simulink model "Drone_Flight_Model_StandAlone_KF_Steady"  (R2016b)
settings: Solver=FixedStepDiscrete  StartTime=0.0  StopTime=20  FixedStep=1/400  RelTol=1e-3  EnableMultiTasking=on
model workspace: external: MAT-File C:\Users\Patrick\Documents\TU\Integration project\AR_Drone_Models\Flight_Models\PD\parameters.mat (data not in the file)
undefined symbols (not defined in the file): accelerometerXyzGains, accelerometerXyzOffsets, Ak, Bk, botCamData, Ck, D_height, D_pitch, D_roll, D_yaw, DiscIntNeverNeededParam, Dk, Drone_StateModeType, dronePowerScaling, g, gyroXyzOffsets, I_height, M, magnetoXyzOffsets, Mass, P_height, P_pitch, P_roll, P_yaw, propDistance, yawTorqueC
libraries: simulink x17, dspstat3 x3, AR_Drone_Sensors x3, AR_Drone_Actuators x3, dspnetwork x2, visionanalysis x2, vrlib x2, AR_Drone_Video x1, AR_Drone_Positioning x1
(part 2 of 2)

== system Drone_Flight_Model_StandAlone_KF_Steady/Sensors, Calibration, Raw state computation/IMU Data Acquisition, Validation, Calibration and Initialization/Sensor Initialization ==
  Measurement_Calculation_Bus : Inport
  Drone_StateModeType : Inport  Port=2
  Bus Creator : BusCreator  Inputs=4
  Bus Selector : BusSelector  OutputSignals=UltraSound_Calculation,AccelNorm_Calculation,Gyro_Calculation,Magnetometer_Calculation
  Gyro Offset Initialization : Subsystem
  Signal Specification : SignalSpecification  SampleTime=1/400
  Initalized Measurement_Calculation_Bus : Outport
  wires:
  Bus Selector/2 -> Bus Creator/2  "<AccelNorm_Calculation>"
  Bus Selector/1 -> Bus Creator/1  "<UltraSound_Calculation>"
  Bus Selector/4 -> Bus Creator/4  "<Magnetometer_Calculation>"
  Measurement_Calculation_Bus/1 -> Bus Selector/1
  Bus Selector/3 -> Gyro Offset Initialization/1(Gyro_Calculation)  "<Gyro_Calculation>"
  Drone_StateModeType/1 -> Gyro Offset Initialization/2(Drone_StateModeType)
  Gyro Offset Initialization/1(Initalized Gyro) -> Bus Creator/3
  Signal Specification/1 -> Initalized Measurement_Calculation_Bus/1
  Bus Creator/1 -> Signal Specification/1

== system Drone_Flight_Model_StandAlone_KF_Steady/Take-Off, Landing, Safety, Motor drivers/AR Drone Motors/MotorMixing ==
  altitude_command : Inport
  roll_command : Inport  Port=2
  pitch_command : Inport  Port=3
  yaw_command : Inport  Port=4
  Constant : Constant  Value=100
  Motor input allocation Result is pure forces : Gain  Gain=[1 1/propDistance 1/propDistance -yawTorqueC; 1 -1/propDistance 1/propDistance yawTorqueC; 1 -1/propDistance -1/propDistance -yawTorqueC; 1 1/propDistance -1/propDistance yawTorqueC]  Multiplication=Matrix(K*u)  ParamDataTypeStr=int16
  Mux1 : Mux
  Newton To PWM : MATLAB Function  TreatAsAtomicUnit=on  mask{dronePowerScaling=dronePowerScaling}
      mask prompts: dronePowerScaling "Drone Power Factor"
  Saturation Dynamic : simulink/Discontinuities/Saturation Dynamic  SCDEnableBlockLinearizationSpecification=on  OutMin=[]  OutMax=[]  OutDataTypeStr=Inherit: Same as second input  OutDataType=fixdt(1, 16)  OutScaling=2^-10  DoSatur=off
  throttleMinimum : Constant  Value=0
  MotorCommands : Outport
  wires:
  pitch_command/1 -> Mux1/3
  roll_command/1 -> Mux1/2
  altitude_command/1 -> Mux1/1
  throttleMinimum/1 -> Saturation Dynamic/3
  Constant/1 -> Saturation Dynamic/1
  Saturation Dynamic/1 -> MotorCommands/1  "rightCommand"
  yaw_command/1 -> Mux1/4
  Newton To PWM/1(PWM) -> Saturation Dynamic/2
  Motor input allocation Result is pure forces/1 -> Newton To PWM/1(thrustIn)
  Mux1/1 -> Motor input allocation Result is pure forces/1

== system Drone_Flight_Model_StandAlone_KF_Steady/Take-Off, Landing, Safety, Motor drivers/Landing//TakeOff Sequence Controller/Landing//TakeOff Altitude Control ==
  Drone StateModeType : Inport
  Attitude Hover Control : Inport  Port=2
  Initialize computation Controller : Subsystem
  Landing Controller : Subsystem
  TakeOff Controller : Subsystem
  Attitude Control : Outport
  wires:
  TakeOff Controller/1(Attitude TakeOff Control) -> Initialize computation Controller/1(Attitude Control)
  Attitude Hover Control/1 -> Landing Controller/1(Hover Control)
  Landing Controller/1(Attitude Landing Control) -> TakeOff Controller/1(Attitude Control)
  Drone StateModeType/1 -> Landing Controller/2(Drone StateModeType), TakeOff Controller/2(Drone StateModeType), Initialize computation Controller/2(Drone StateModeType)
  Initialize computation Controller/1(Initialization Control) -> Attitude Control/1

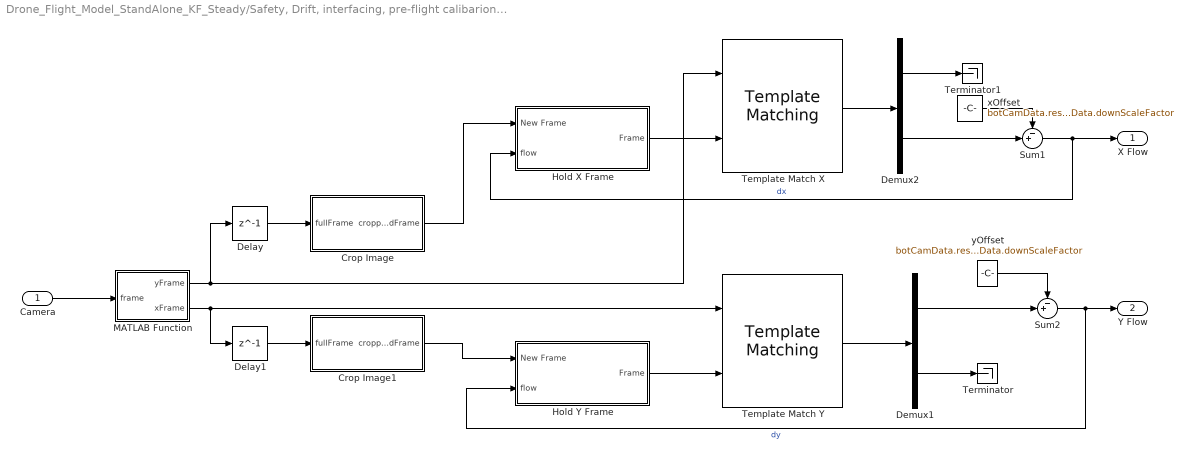
== system Drone_Flight_Model_StandAlone_KF_Steady/Safety, Drift, interfacing, pre-flight calibarion/Optical Flow/Optical Flow/Template Matching ==
  Camera : Inport
  Crop Image : MATLAB Function  TreatAsAtomicUnit=on
  Crop Image1 : MATLAB Function  TreatAsAtomicUnit=on
  Delay : Delay  DelayLength=1
  Delay1 : Delay  DelayLength=1
  Demux1 : Demux  Outputs=2
  Demux2 : Demux  Outputs=2
  Hold X Frame : Subsystem
  Hold Y Frame : Subsystem
  MATLAB Function : MATLAB Function  TreatAsAtomicUnit=on
  Sum1 : Sum  Inputs=-+|  AccumDataTypeStr=double  OutDataTypeStr=double
  Sum2 : Sum  Inputs=-+|  AccumDataTypeStr=double  OutDataTypeStr=double
  Template Match X : visionanalysis/Template Matching  metric=Sum of absolute differences  output=Best match location  method=Three-step  nMetric=off  nSize=3  roi=off  roiValid=off  accumMode=Binary point scaling  accumWordLength=32  accumFracLength=0  prodOutputMode=Binary point scaling  prodOutputWordLength=32  prodOutputFracLength=0  roundingMode=Floor  overflowMode=off
  Template Match Y : visionanalysis/Template Matching  metric=Sum of absolute differences  output=Best match location  method=Three-step  nMetric=off  nSize=3  roi=off  roiValid=off  accumMode=Binary point scaling  accumWordLength=32  accumFracLength=0  prodOutputMode=Binary point scaling  prodOutputWordLength=32  prodOutputFracLength=0  roundingMode=Floor  overflowMode=off
  Terminator : Terminator
  Terminator1 : Terminator
  xOffset : Constant  Value=botCamData.resolution(2)/2/botCamData.downScaleFactor
  yOffset : Constant  Value=botCamData.resolution(1)/2/botCamData.downScaleFactor
  X Flow : Outport
  Y Flow : Outport  Port=2
  wires:
  Demux1/2 -> Terminator/1
  Demux2/1 -> Terminator1/1
  Sum2/1 -> Y Flow/1, Hold Y Frame/2(flow)  "dy"
  Hold Y Frame/1(Frame) -> Template Match Y/2
  Demux1/1 -> Sum2/2
  Template Match Y/1 -> Demux1/1
  MATLAB Function/1(yFrame) -> Template Match X/1, Delay/1
  Delay/1 -> Crop Image/1(fullFrame)
  yOffset/1 -> Sum2/1
  Crop Image/1(croppedFrame) -> Hold X Frame/1(New Frame)
  xOffset/1 -> Sum1/1
  Demux2/2 -> Sum1/2
  Template Match X/1 -> Demux2/1
  Hold X Frame/1(Frame) -> Template Match X/2
  Sum1/1 -> X Flow/1, Hold X Frame/2(flow)  "dx"
  Camera/1 -> MATLAB Function/1(frame)
  Delay1/1 -> Crop Image1/1(fullFrame)
  MATLAB Function/2(xFrame) -> Delay1/1, Template Match Y/1
  Crop Image1/1(croppedFrame) -> Hold Y Frame/1(New Frame)

== system Drone_Flight_Model_StandAlone_KF_Steady/Safety, Drift, interfacing, pre-flight calibarion/Optical Flow/Optical Flow Reset/Drone_StateMode Reset Condition ==
  Drone_StateMode : Inport
  Enumerated Constant2 : simulink/Sources/Enumerated Constant  OutDataTypeStr=Enum: Drone_StateModeType  Value=Drone_StateModeType.Drift_Compensated_Flight  SampleTime=inf
      settings: AttributesFormatString=%<Value>
  Offset Calc Reset Boolean : RelationalOperator  Operator=~=  OutDataTypeStr=boolean  RndMeth=Nearest
  Drone_StateMode Reset : Outport
  wires:
  Drone_StateMode/1 -> Offset Calc Reset Boolean/1
  Enumerated Constant2/1 -> Offset Calc Reset Boolean/2
  Offset Calc Reset Boolean/1 -> Drone_StateMode Reset/1

== system Drone_Flight_Model_StandAlone_KF_Steady/Safety, Drift, interfacing, pre-flight calibarion/Optical Flow/Optical Flow Reset/PQR Reset Condition ==
  PQR : Inport
  Abs : Abs
  Demux : Demux  Outputs=3
  Logical Operator : Logic  Operator=OR  Inputs=3  AllPortsSameDT=off  OutDataTypeStr=boolean
  Max P : simulink/Logic and Bit Operations/Compare To Constant  relop=>  const=30  OutDataTypeStr=uint8
  Max Q : simulink/Logic and Bit Operations/Compare To Constant  relop=>  const=30  OutDataTypeStr=uint8
  Max R : simulink/Logic and Bit Operations/Compare To Constant  relop=>  const=30  OutDataTypeStr=uint8
  PQR Reset : Outport
  wires:
  Demux/1 -> Max P/1
  Demux/2 -> Max Q/1
  Max P/1 -> Logical Operator/1
  Max Q/1 -> Logical Operator/2
  Logical Operator/1 -> PQR Reset/1
  Demux/3 -> Max R/1
  Max R/1 -> Logical Operator/3
  Abs/1 -> Demux/1
  PQR/1 -> Abs/1

== system Drone_Flight_Model_StandAlone_KF_Steady/Safety, Drift, interfacing, pre-flight calibarion/Optical Flow/Optical Flow Reset/Zdot Reset condition ==
  Z Zdot : Inport
  Abs : Abs
  Demux : Demux  Outputs=2
  Max Zdot : simulink/Logic and Bit Operations/Compare To Constant  relop=>  const=20  OutDataTypeStr=uint8
  Smooth Height : DiscreteTransferFcn  Numerator=[0.05]  Denominator=[1 -0.95]
  Terminator : Terminator
  Zdot Reset : Outport
  wires:
  Max Zdot/1 -> Zdot Reset/1
  Z Zdot/1 -> Demux/1
  Abs/1 -> Smooth Height/1
  Demux/1 -> Terminator/1
  Demux/2 -> Abs/1
  Smooth Height/1 -> Max Zdot/1

== system Drone_Flight_Model_StandAlone_KF_Steady/Sensors, Calibration, Raw state computation/IMU Data Acquisition, Validation, Calibration and Initialization/Measurement Verification and Calibration/Measurement calibration correction ==
  note: Cannot measure below ~15cm so it is set as minimum
  MeasurementDataBus : Inport
  Accelerometer calibration : Subsystem
  Bus Creator1 : BusCreator  Inputs=4
  Bus Selector : BusSelector  OutputSignals=Ultrasound_Measure,Accelerometer_Measure,BodyRates_Measure,Magnetometer_Measure
  Calibration_Scale_and_Offset1 : Subsystem
  Gyro offset : Subsystem
  Height Lookup Table : Lookup_n-D  NumberOfTableDimensions=1  BreakpointsForDimension1="[880\t896.633239612621\t926.474851608872\t963.444876423216\t1026.24093976506\t1108.89023120183\t1201.82715535194\t1299.73045340950\t1400.50546704155\t1505.69346105789\t1616.54602249063\t1723.41949303820\t1829.85256143274\t1941.57919400187\t2209.22354901416\t2928.85067166510\t3648.07466416745\t4365.64658835291\t5080.81671757845\t5793.22994251437\t6544.72960690752\t7259.40674789128\t8002\t8664.09897525619\t9309.60334916271\t9993]"  Table="[15\t20\t23\t26\t29\t32\t35\t38\t41\t44\t47\t50\t53\t56\t63\t83\t103\t123\t143\t163\t183\t203\t223\t243\t263\t283]"  InternalRulePriority=Speed  RndMeth=Simplest  InputSameDT=on
  MATLAB Function : MATLAB Function  TreatAsAtomicUnit=on
  Measurement_Calculation_Bus : Outport
  wires:
  Bus Selector/1 -> MATLAB Function/1(Ultrasound_Measure)  "<Ultrasound_Measure>"
  Gyro offset/1(Gyro Offset Remove) -> Bus Creator1/3  "Gyro_Calculation"
  Bus Selector/2 -> Accelerometer calibration/1(Accel)  "<Accelerometer_Measure>"
  Accelerometer calibration/1(Accel_Norm) -> Bus Creator1/2  "AccelNorm_Calculation"
  Height Lookup Table/1 -> Bus Creator1/1  "UltraSound_Calculation"
  Calibration_Scale_and_Offset1/1(Normalized  Magnetometer) -> Bus Creator1/4  "Magnetometer_Calculation"
  MeasurementDataBus/1 -> Bus Selector/1
  Bus Selector/3 -> Gyro offset/1(Raw Gyro Values)  "<BodyRates_Measure>"
  Bus Creator1/1 -> Measurement_Calculation_Bus/1
  Bus Selector/4 -> Calibration_Scale_and_Offset1/1(RawMag)  "<Magnetometer_Measure>"
  MATLAB Function/1(processed_Ultrasound) -> Height Lookup Table/1  "UltraSound_Calculation"

== system Drone_Flight_Model_StandAlone_KF_Steady/Sensors, Calibration, Raw state computation/IMU Data Acquisition, Validation, Calibration and Initialization/Sensor Initialization/Gyro Offset Initialization ==
  note: Gyro Offset Initialization
      | The gyro is calibrated each time before flight takes place during the
      | Drone_StateModeType.Initialize state. The gyro is the only sensor that
      | can be re calibrated from the static take off position.
  Gyro_Calculation : Inport
  Drone_StateModeType : Inport  Port=2
  Add : Sum  Inputs=+-
  Compute Gyro Offset : dspstat3/Mean  run=on  reset_popup=Rising edge  directionMode=Each column  dimension=1  roiEnable=off  roiType=Rectangles  roiPortion=Entire ROI  roiOutput=Individual statistics for each ROI  roiFlag=off  outputDataTypeStr=Inherit: Same as accumulator  outputLastDataTypeStr=Inherit: Same as accumulator  outputMin=[]  outputMax=[]  roundingMode=Floor  overflowMode=off
  Enumerated Constant2 : simulink/Sources/Enumerated Constant  OutDataTypeStr=Enum: Drone_StateModeType  Value=Drone_StateModeType.Initialize_Sensors  SampleTime=inf
      settings: AttributesFormatString=%<Value>
  Offset Calc Reset Boolean : RelationalOperator  Operator===  OutDataTypeStr=boolean  RndMeth=Nearest
  Offset Memory : Memory  InheritSampleTime=on
  Output Selector : Switch  Criteria=u2 > Threshold
  Output Selector Reset Boolean : RelationalOperator  Operator=~=  OutDataTypeStr=boolean  RndMeth=Nearest
  Initalized Gyro : Outport
  wires:
  Offset Calc Reset Boolean/1 -> Compute Gyro Offset/2
  Gyro_Calculation/1 -> Add/1, Compute Gyro Offset/1
  Output Selector Reset Boolean/1 -> Output Selector/2
  Compute Gyro Offset/1 -> Output Selector/3
  Output Selector/1 -> Offset Memory/1, Add/2
  Add/1 -> Initalized Gyro/1  "Gyro_Calculation"
  Drone_StateModeType/1 -> Output Selector Reset Boolean/2, Offset Calc Reset Boolean/2
  Offset Memory/1 -> Output Selector/1
  Enumerated Constant2/1 -> Output Selector Reset Boolean/1, Offset Calc Reset Boolean/1

== system Drone_Flight_Model_StandAlone_KF_Steady/Take-Off, Landing, Safety, Motor drivers/Landing//TakeOff Sequence Controller/Landing//TakeOff Altitude Control/Initialize computation Controller ==
  note: Magnetometer initialization controls
      | The motors influence the magnetometer measurement.
      | The motors are set to turn at low RPM while computing the yaw offset.
  Attitude Control : Inport
  Drone StateModeType : Inport  Port=2
  Enumerated Constant2 : simulink/Sources/Enumerated Constant  OutDataTypeStr=Enum: Drone_StateModeType  Value=Drone_StateModeType.Initialize_Computation  SampleTime=inf
      settings: AttributesFormatString=%<Value>
  Initialize Boolean : RelationalOperator  Operator=~=  OutDataTypeStr=boolean  RndMeth=Nearest
  Magneto initialization thrust : Constant  Value="Mass * 9.81 * 0.15  / 4"
  Switch2 : Switch  Criteria=u2 > Threshold
  Initialization Control : Outport
  wires:
  Enumerated Constant2/1 -> Initialize Boolean/1
  Drone StateModeType/1 -> Initialize Boolean/2
  Attitude Control/1 -> Switch2/1
  Initialize Boolean/1 -> Switch2/2
  Switch2/1 -> Initialization Control/1
  Magneto initialization thrust/1 -> Switch2/3

== system Drone_Flight_Model_StandAlone_KF_Steady/Take-Off, Landing, Safety, Motor drivers/Landing//TakeOff Sequence Controller/Landing//TakeOff Altitude Control/Landing Controller ==
  note: Landing Sequence control
      | The last known altitude PWM signal is decayed such that the drone loses altitude controlled.
  Hover Control : Inport
  Drone StateModeType : Inport  Port=2
  Decay Gain : Gain  Gain=0.9992
  Enumerated Constant1 : simulink/Sources/Enumerated Constant  OutDataTypeStr=Enum: Drone_StateModeType  Value=Drone_StateModeType.Landing_RampDown  SampleTime=inf
      settings: AttributesFormatString=%<Value>
  Landing Boolean : RelationalOperator  Operator=~=  OutDataTypeStr=boolean  RndMeth=Nearest
  Memory : Memory
  Switch1 : Switch  Criteria=u2 > Threshold
  Attitude Landing Control : Outport
  wires:
  Memory/1 -> Decay Gain/1
  Landing Boolean/1 -> Switch1/2
  Decay Gain/1 -> Switch1/3
  Enumerated Constant1/1 -> Landing Boolean/1
  Hover Control/1 -> Switch1/1
  Switch1/1 -> Memory/1, Attitude Landing Control/1
  Drone StateModeType/1 -> Landing Boolean/2

== system Drone_Flight_Model_StandAlone_KF_Steady/Take-Off, Landing, Safety, Motor drivers/Landing//TakeOff Sequence Controller/Landing//TakeOff Altitude Control/TakeOff Controller ==
  note: Take Off control
      | The altitude PWM signal is ramped up from a bottom value to a maximum of 45% of hover thrust before
      | height control is enabled.
  Attitude Control : Inport
  Drone StateModeType : Inport  Port=2
  Base Required Thrust Per Motor [N] : Constant  Value=Mass * 9.81 * 0.45 / 4
  Discrete-Time Integrator : DiscreteIntegrator  gainval=1  ExternalReset=level  InitialConditionSource=external  InitialConditionSetting=State (most efficient)  SampleTime=-1  ICPrevOutput=DiscIntNeverNeededParam  ICPrevScaledInput=DiscIntNeverNeededParam
  Enumerated Constant2 : simulink/Sources/Enumerated Constant  OutDataTypeStr=Enum: Drone_StateModeType  Value=Drone_StateModeType.Take_Off  SampleTime=inf
      settings: AttributesFormatString=%<Value>
  Initial Thrust value : Constant  Value="Mass * 9.81 * 0.2  / 4"
  Saturation : Saturate  UpperLimit=0.5*Mass * 9.81 / 4  LowerLimit=0
  Switch2 : Switch  Criteria=u2 > Threshold
  TakeOff Boolean : RelationalOperator  Operator=~=  OutDataTypeStr=boolean  RndMeth=Nearest
  Attitude TakeOff Control : Outport
  wires:
  Enumerated Constant2/1 -> TakeOff Boolean/1
  Saturation/1 -> Switch2/3
  Drone StateModeType/1 -> TakeOff Boolean/2
  Attitude Control/1 -> Switch2/1
  TakeOff Boolean/1 -> Switch2/2, Discrete-Time Integrator/2
  Switch2/1 -> Attitude TakeOff Control/1
  Discrete-Time Integrator/1 -> Saturation/1
  Base Required Thrust Per Motor [N]/1 -> Discrete-Time Integrator/1
  Initial Thrust value/1 -> Discrete-Time Integrator/3

== system Drone_Flight_Model_StandAlone_KF_Steady/Safety, Drift, interfacing, pre-flight calibarion/Optical Flow/Optical Flow/Template Matching/Hold X Frame ==
  New Frame : Inport
  flow : Inport  Port=2
  Delay2 : Delay  DelayLength=1  InitialConditionSource=Input port
      settings: InputPortMap=u0,p4
  Delay3 : Delay  DelayLength=1
  MATLAB Function : MATLAB Function  TreatAsAtomicUnit=on
  Frame : Outport
  wires:
  Delay2/1 -> MATLAB Function/2(heldFrame)
  MATLAB Function/1(referenceFrame) -> Delay2/1, Frame/1
  New Frame/1 -> MATLAB Function/1(currentFrame), Delay2/2
  flow/1 -> Delay3/1
  Delay3/1 -> MATLAB Function/3(flow)

== system Drone_Flight_Model_StandAlone_KF_Steady/Safety, Drift, interfacing, pre-flight calibarion/Optical Flow/Optical Flow/Template Matching/Hold Y Frame ==
  New Frame : Inport
  flow : Inport  Port=2
  Delay2 : Delay  DelayLength=1  InitialConditionSource=Input port
      settings: InputPortMap=u0,p4
  Delay3 : Delay  DelayLength=1
  MATLAB Function : MATLAB Function  TreatAsAtomicUnit=on
  Frame : Outport
  wires:
  Delay2/1 -> MATLAB Function/2(heldFrame)
  MATLAB Function/1(referenceFrame) -> Delay2/1, Frame/1
  New Frame/1 -> MATLAB Function/1(currentFrame), Delay2/2
  flow/1 -> Delay3/1
  Delay3/1 -> MATLAB Function/3(flow)

== system Drone_Flight_Model_StandAlone_KF_Steady/Sensors, Calibration, Raw state computation/IMU Data Acquisition, Validation, Calibration and Initialization/Measurement Verification and Calibration/Measurement calibration correction/Accelerometer calibration ==
  Accel : Inport
  Apply calibration parameters : Subsystem
  Data Type Conversion : DataTypeConversion  OutDataTypeStr=double
  Normalize Vector : vrlib/Utilities/Normalize Vector  Commented=through  maxzero=0
  Accel_Norm : Outport
  wires:
  Accel/1 -> Data Type Conversion/1
  Data Type Conversion/1 -> Apply calibration parameters/1(Raw Accelerometer Data)
  Normalize Vector/1 -> Accel_Norm/1
  Apply calibration parameters/1(Calibrated Accelerometer Data) -> Normalize Vector/1

== system Drone_Flight_Model_StandAlone_KF_Steady/Sensors, Calibration, Raw state computation/IMU Data Acquisition, Validation, Calibration and Initialization/Measurement Verification and Calibration/Measurement calibration correction/Calibration_Scale_and_Offset1 ==
  RawMag : Inport
  Add : Sum  Inputs=-+
  Constant : Constant  Value=magnetoXyzOffsets
  Normalize Vector : vrlib/Utilities/Normalize Vector  maxzero=0
  Normalized  Magnetometer : Outport
  wires:
  Add/1 -> Normalize Vector/1
  Constant/1 -> Add/1
  Normalize Vector/1 -> Normalized  Magnetometer/1
  RawMag/1 -> Add/2

== system Drone_Flight_Model_StandAlone_KF_Steady/Sensors, Calibration, Raw state computation/IMU Data Acquisition, Validation, Calibration and Initialization/Measurement Verification and Calibration/Measurement calibration correction/Gyro offset ==
  Raw Gyro Values : Inport
  Constant : Constant  Value=gyroXyzOffsets  VectorParams1D=off
  Demux : Demux  Outputs=3
  Demux1 : Demux  Outputs=3
  Mux1 : Mux  Inputs=3
  Process Raw Rate Gyro Data : Subsystem
  Sum : Sum  Inputs=|+-
  Sum1 : Sum  Inputs=|+-
  Sum2 : Sum  Inputs=|+-
  Gyro Offset Remove : Outport
  wires:
  Demux/3 -> Sum2/1
  Sum1/1 -> Mux1/2
  Demux1/1 -> Sum/2
  Sum2/1 -> Mux1/3
  Demux/2 -> Sum1/1
  Demux/1 -> Sum/1
  Sum/1 -> Mux1/1
  Mux1/1 -> Process Raw Rate Gyro Data/1(Raw Rate Gyro Data)
  Demux1/2 -> Sum1/2
  Demux1/3 -> Sum2/2
  Process Raw Rate Gyro Data/1(Processed Data) -> Gyro Offset Remove/1
  Constant/1 -> Demux1/1
  Raw Gyro Values/1 -> Demux/1

== system Drone_Flight_Model_StandAlone_KF_Steady/Sensors, Calibration, Raw state computation/IMU Data Acquisition, Validation, Calibration and Initialization/Measurement Verification and Calibration/Measurement calibration correction/Accelerometer calibration/Apply calibration parameters ==
  Raw Accelerometer Data : Inport
  Acclerometer Calibration Gains : Constant  Value=accelerometerXyzGains
  Acclerometer Calibration Offsets : Constant  Value=accelerometerXyzOffsets
  Add : Sum  Inputs=+-
  Divide : Product  Inputs=*/
  Calibrated Accelerometer Data : Outport
  wires:
  Divide/1 -> Calibrated Accelerometer Data/1
  Raw Accelerometer Data/1 -> Add/1
  Acclerometer Calibration Gains/1 -> Divide/2
  Acclerometer Calibration Offsets/1 -> Add/2
  Add/1 -> Divide/1

== system Drone_Flight_Model_StandAlone_KF_Steady/Sensors, Calibration, Raw state computation/IMU Data Acquisition, Validation, Calibration and Initialization/Measurement Verification and Calibration/Measurement calibration correction/Gyro offset/Process Raw Rate Gyro Data ==
  note: const float Sensitivity[ 3 ] = { 0.0609 , 0.0609 , 0.0609 } ;
  Raw Rate Gyro Data : Inport
  Flip Pitch Yaw Direction For Calculation #235 : Gain  Gain=[1 -1 -1]
  Gain : Gain  Gain=[0.0609, 0.0609, 0.0609]  ParamDataTypeStr=double
  Processed Data : Outport
  wires:
  Raw Rate Gyro Data/1 -> Gain/1
  Flip Pitch Yaw Direction For Calculation #235/1 -> Processed Data/1
  Gain/1 -> Flip Pitch Yaw Direction For Calculation #235/1

== matlab function Drone_Flight_Model_StandAlone_KF_Steady/Safety, Drift, interfacing, pre-flight calibarion/Downscaled Bottom Camera/Downscale Chroma Image ==
  data: YCbCr422In input; cameraChroma output; width parameter; height parameter; downScaleFactor parameter
function cameraChroma    = downscaleY(YCbCr422In,width, height, downScaleFactor)
 
cameraChroma = uint8(zeros(height/downScaleFactor,width/downScaleFactor));
if ~isempty(YCbCr422In)

    %% Downsample and keep only the chromatic value

    for verticalIndex = 1 : 1 : height/downScaleFactor;             % indexing for downsampled vertical direction
        for horizontalIndex = 1 : 1 : (width / 2)/downScaleFactor;  % indexing for downsampled horizontal direction
            index = 4 * (downScaleFactor * (verticalIndex - 1) * (width / 2) + downScaleFactor * horizontalIndex) - 3;  % translate the horizontal and vertical indexes into the index into the video input
            cameraChroma(verticalIndex, 2 * horizontalIndex - [1 0]) = [YCbCr422In(index+1) YCbCr422In(index+3)];
        end
    end
end
end

== matlab function Drone_Flight_Model_StandAlone_KF_Steady/Safety, Drift, interfacing, pre-flight calibarion/Optical Flow/Optical Flow/Template Matching/Crop Image ==
  data: fullFrame input; croppedFrame output
function croppedFrame = CropImage(fullFrame)

%% Template matching works by pixel shifting a smaller image within the full image
% Exhaustive template matching will compute all possible pixel shifts.
% Because of this the cropAmount influences the computation time
% quadratically. A small crop amount increases the computation speed but
% also limits the maximum detectable pixel shift between frames. 
% Three step template matching also has increasing computational time with
% increasing cropAmount, but much less so than the exhaustive method.
cropAmount = 7;
%% Maximizing camera FPS
% Doubling the camera FPS doubles the computation time but also means you 
% can halve the cropAmount and still detect the same velocity range, which 
% reduces the computational time up to a factor 4.
%% FPS limitations
% Using a very high fps means that slow drone movements will not lead to
% significant enough displacement between images. This means that slow
% drift is not detected. Holding the reference frame untill movement is
% deteced is a way around this.


[row, col] = size(fullFrame);
croppedFrame = fullFrame(1 + cropAmount : row - cropAmount, 1 + cropAmount : col - cropAmount);
% croppedFrame = fullFrame(1 + cropAmount : row - cropAmount, 1 : col);

== stateflow chart Drone_Flight_Model_StandAlone_KF_Steady/Safety, Drift, interfacing, pre-flight calibarion/Supervisory Flight Controller ==
  state stateChecks [parallel]
    settings: executionOrder=1
    note: Description:
        | This state containts the sub states used to detect specific operating conditions
    state batteryFaultCheck [parallel]
      settings: executionOrder=1
      note: Description:
          | This state will indicate whether the battery has enough voltage.
      state batteryNominal
      state batteryLow
      batteryLow -> batteryNominal : [Measured_Battery_Voltage>=10.6]
      batteryNominal -> batteryLow : [Measured_Battery_Voltage<10.6]
      (default) -> batteryLow
    state orientationFaultCheck [parallel]
      settings: executionOrder=2
      note: Description:
          | This state will indicate whether the drone is in a safe orientation
      state nominalOrientation
      state unsafeOrientation
      unsafeOrientation -> nominalOrientation : [all(abs(Euler_Angles(1:2)) < 35)]
      nominalOrientation -> unsafeOrientation : [any(abs(Euler_Angles(1:2)) >= 35)]
      (default) -> unsafeOrientation
    state safeHeightCheck [parallel]
      settings: executionOrder=3
      note: Description:
          | This state will indicate whether the drone is close enough to the groudn for the final landing procedure
      state safeLandingHeight
      state unsafeLandingHeight
      unsafeLandingHeight -> safeLandingHeight : [Altitude < 25]
      safeLandingHeight -> unsafeLandingHeight : [Altitude > 30]
      (default) -> unsafeLandingHeight
  state Drone_State [parallel]
    settings: executionOrder=2
    note: Description:
        | This state contains the logic governing the drone behaviour based on user input and drone state checks
    state WaitForHost
    state Initialize_Sensors
    state Initialize_Computation
    state Take_Off
    state Drift_Compensated_Flight
    state Landing_Terminate
    state Landing_RampDown
    state Landing_Descent
    (default) -> WaitForHost
    Landing_Terminate -> WaitForHost : [ (hostCmd == Drone_StateModeType.WaitForHost)]
    WaitForHost -> Initialize_Sensors : [ (hostCmd == Drone_StateModeType.Drift_Compensated_Flight)...
        | && in(stateChecks.batteryFaultCheck.batteryNominal)...
        | && in (stateChecks.orientationFaultCheck.nominalOrientation)...
        | && after(1.5,sec)]
    Initialize_Sensors -> Initialize_Computation : [after(0.5,sec)]
    Initialize_Computation -> Take_Off : [after(3,sec)]
    Take_Off -> Landing_Terminate [order 2] : [(hostCmd == Drone_StateModeType.Landing_Terminate)]
    Take_Off -> Drift_Compensated_Flight [order 1] : [after(2,sec)]
    Drift_Compensated_Flight -> Landing_Descent [order 1] : [(hostCmd == Drone_StateModeType.Landing_Descent)...
        | ||in(stateChecks.batteryFaultCheck.batteryLow) ]
    Drift_Compensated_Flight -> Landing_Terminate [order 2] : [in(stateChecks.orientationFaultCheck.unsafeOrientation)...
        | ||(hostCmd == Drone_StateModeType.Landing_Terminate)]
    Landing_RampDown -> Landing_Terminate : [after(2.0,sec)...
        | ||(hostCmd == Drone_StateModeType.Landing_Terminate)]
    Landing_Descent -> Landing_RampDown [order 1] : [in(stateChecks.safeHeightCheck.safeLandingHeight)]
    Landing_Descent -> Landing_Terminate [order 2] : [(hostCmd == Drone_StateModeType.Landing_Terminate)]
  data: hostCmd input Enum: Drone_StateModeType; Drone_StateMode output Enum: Drone_StateModeType; Measured_Battery_Voltage input; Euler_Angles input; Altitude input
  data hostCmd settings: description=|
      | The hostCmd can take the values 0,1 and 2.
      | 
      | 0 - default state when the drone is powered up.
      | 1 - Takeoff
      | 2 - Landing

== matlab function Drone_Flight_Model_StandAlone_KF_Steady/Safety, Drift, interfacing, pre-flight calibarion/Drone TO PC UDP IO/Gather Data and transfer rates/MATLAB Function1 ==
  data: dataIn input; combinedData output
function combinedData = combineMultipleSamples(dataIn)

persistent storedData
if isempty(storedData)
    storedData = zeros(66,1);
end
storedData(1:33) = storedData(34:66);
storedData(34:66) = dataIn;
combinedData = storedData;

== matlab function Drone_Flight_Model_StandAlone_KF_Steady/Sensors, Calibration, Raw state computation/Unwrap Yaw Angle/MATLAB Function ==
  data: wrappedYaw input; unwrappedYaw output; previousYaw input
function unwrappedYaw = unwrapYaw(wrappedYaw, previousYaw)
%#codegen

persistent offset
if isempty(offset)
   offset = 0; 
end

threshold = 150;

% check if the yaw switched from ~180 to ~-180
if (previousYaw > threshold && wrappedYaw < -threshold)
    offset = offset + 360;
end

% check if the yaw switched from ~-180 to ~180
if (previousYaw < -threshold && wrappedYaw > threshold)
    offset = offset - 360;
end

unwrappedYaw = wrappedYaw + offset;

== matlab function Drone_Flight_Model_StandAlone_KF_Steady/Controller/Zdot transform/Rotation matrix/Rotm in euler ==
  data: alpha input size=3,1; Rbv output size=3,3
function Rbv = fcn(alpha)
Rbv = [1,0,0;0,cos(alpha(1)),sin(alpha(1));0,-sin(alpha(1)),cos(alpha(1))]*...
      [cos(alpha(2)),0,-sin(alpha(2));0,1,0;sin(alpha(2)),0,cos(alpha(2))]*...
      [cos(alpha(3)),sin(alpha(3)),0;-sin(alpha(3)),cos(alpha(3)),0;0,0,1];

== matlab function Drone_Flight_Model_StandAlone_KF_Steady/Sensors, Calibration, Raw state computation/Calculate Roll Pitch/MATLAB Function ==
  data: Ax_Ay_Az input; Roll output; Pitch output
function [Roll,Pitch] = CalculateAngle(Ax_Ay_Az)

Pitch = atan( Ax_Ay_Az(1) / sqrt( Ax_Ay_Az(2)^2 + Ax_Ay_Az(3)^2));
Roll = atan( Ax_Ay_Az(2) / sqrt( Ax_Ay_Az(1)^2 + Ax_Ay_Az(3)^2));

== matlab function Drone_Flight_Model_StandAlone_KF_Steady/Safety, Drift, interfacing, pre-flight calibarion/Optical Flow/Optical Flow/Template Matching/MATLAB Function ==
  data: yFrame output; frame input; xFrame output
function [yFrame, xFrame] = downSampleFrames(frame)

xFrame = frame(1:4:end,:);
yFrame = frame(:,1:4:end);

== matlab function Drone_Flight_Model_StandAlone_KF_Steady/Safety, Drift, interfacing, pre-flight calibarion/Optical Flow/Optical Flow/Template Matching/Hold Y Frame/MATLAB Function ==
  data: currentFrame input uint8; referenceFrame output; heldFrame input uint8; flow input
function referenceFrame  = holdFrame(currentFrame,heldFrame,flow)

%% This MATLAB function block holds the T frame untill movement is detected
% If the T frame were updated every step, slow movements would not be
% registered. By holding the frame movement can be measured over multiple
% frames.

if (flow ==0)
    referenceFrame = heldFrame;
else
    referenceFrame = currentFrame;
end

== matlab function Drone_Flight_Model_StandAlone_KF_Steady/Safety, Drift, interfacing, pre-flight calibarion/Optical Flow/Optical Flow/Scale Optical Flow Steps ==
  data: xFlow input; xPos output; yFlow input; zPos input; yPos output; downScaleFactor parameter; FOV parameter
function [xPos, yPos] = scaleOpticalFlow(xFlow,yFlow,zPos,downScaleFactor,FOV)
xFOV = FOV * 0.75 / 180 * pi;
yFOV = FOV / 180 * pi;

% prevent division by zero when zPos = 0 -> xMax,xMin,yMax,yMin = 0
if zPos > 0 
    xMin = - tan(xFOV/2) * zPos;
    xMax = tan(xFOV/2) * zPos;
    yMin = - tan(yFOV/2) * zPos;
    yMax = tan(yFOV/2) * zPos;

    xResolution = 240/downScaleFactor;
    yResolution = 320/downScaleFactor;

    %determine how many real world cm one camera pixel is
    xScale = xResolution / (xMax - xMin);
    yScale = yResolution / (yMax - yMin);
    
    %scale the optical flow components
    xPos = xFlow / xScale;
    yPos = - yFlow / yScale; % direction is reversed

else
   xPos = 0;
   yPos = 0;
end

== matlab function Drone_Flight_Model_StandAlone_KF_Steady/Sensors, Calibration, Raw state computation/Compute Yaw ==
  data: Roll input; Pitch input; Magneto input; Yaw output
function Yaw = computeYaw(Roll, Pitch, Magneto)

% convert to rad for calculation
Roll = Roll / 360 * 2 * pi;
Pitch = Pitch / 360 * 2 * pi;

% Applications of Magnetic Sensors for Low Cost Compass Systems, Michael J. Caruso, Honeywell, SSEC.
% Magneto(3) sign is switched as we define the z axis as positive up.

var1 = Magneto(2)*cos(Roll)-Magneto(3)*sin(Roll);
var2 = Magneto(1)*cos(Pitch)+Magneto(2)*sin(Pitch)*sin(Roll)+Magneto(3)*cos(Roll)*sin(Pitch);

% scale to [-180 180] deg
Yaw = - atan2(var1,var2) * 180 / pi;

== matlab function Drone_Flight_Model_StandAlone_KF_Steady/Safety, Drift, interfacing, pre-flight calibarion/Drone TO PC UDP IO/Gather Data and transfer rates/Encode Outgoing Packets ==
  data: droneStateMode input; message output; batteryLevel input; roll input; pitch input; yaw input; altitude input; motorCmd input; flags input
function message = packageEncode(droneStateMode, batteryLevel, roll, pitch, yaw, altitude, motorCmd, flags)

persistent checksum
if isempty(checksum)
    checksum = uint8(0);
end

%% Generate a tick/checksum

if checksum < uint8(255)
    checksum = uint8(checksum + 1);
else
    checksum  = uint8(0);
end

%% The message format is:
% Checksum          uint8[1]
% BatterlyLevel     single[1] cast as uint8[4] 
% DroneStateMode    DroneStateModeType[1] cast as uint8[1]
% Roll              single[1] cast as uint8[4] 
% Pitch             single[1] cast as uint8[4] 
% Yaw               single[1] cast as uint8[4] 
% Altitude          single[1] cast as uint8[4] 
% Motor             single[4] cast as uint8[16]
% chkSum&Reset flag uint8[2]
% Target data       single[15] cast as uint8[60]
% Extra data        single[1] cast as uint8[4] 

%% Cast data to a single before typecasting to uint8
stateModeMessage = uint8(droneStateMode);
batteryMessage = typecast(single(batteryLevel),'uint8');
rollMessage = typecast(single(roll),'uint8');
pitchMessage = typecast(single(pitch),'uint8');
yawMessage = typecast(single(yaw),'uint8');
altitudeMessage = typecast(single(altitude),'uint8');
motorMessage = typecast(single(motorCmd),'uint8');
flagsMessage = uint8(flags);


%% Combine into a message
message = uint8(zeros(1,40));
message(1) = checksum;
message(2:5) = batteryMessage;
message(6) = stateModeMessage;
message(7:10) = rollMessage;
message(11:14) = pitchMessage;
message(15:18) = yawMessage;
message(19:22) = altitudeMessage;
message(23:38) = motorMessage;
message(39:40) = flagsMessage;
% message = [checksum batteryMessage stateModeMessage dataMessage];

== matlab function Drone_Flight_Model_StandAlone_KF_Steady/Safety, Drift, interfacing, pre-flight calibarion/Drone TO PC UDP IO/Decode Incoming Packets ==
  data: message input; length input; userCommand output Enum: Drone_StateModeType; maxUpdateDelay parameter; ledColor output; enableTracking output; remoteControl output; trimCommands output
function [userCommand, ledColor, enableTracking, remoteControl, trimCommands]  = packageDecode(message, length, maxUpdateDelay)

persistent lastReceivedTick updatesSinceLastTick ledCounter lastUserCommand savedTrimCommands savedEnableTracking;
if isempty(lastReceivedTick) || isempty(updatesSinceLastTick) || isempty(ledCounter) ...
       || isempty(lastUserCommand) || isempty(savedTrimCommands)
    lastReceivedTick = 0;
    updatesSinceLastTick = 0;
    ledCounter = 0;
    %% Initial state = WaitForHost
    lastUserCommand = Drone_StateModeType(1);
    savedTrimCommands = int8([0 0]);
    savedEnableTracking = uint8(0);
end;

% default return: use last user command
userCommand = lastUserCommand;
ledColor = 2;
enableTracking = savedEnableTracking;
remoteControl = uint8(0);
trimCommands = savedTrimCommands;

% check if a message is received
if length == 6
   % decode message
   newTick = double(message(1));
   newUserCommand = Drone_StateModeType(message(2));
   enableTracking = message(3);
   remoteControl = message(4);
   trimCommands(1) = typecast(message(5),'int8');
   trimCommands(2) = typecast(message(6),'int8');
   if newTick ~= lastReceivedTick
       % If this is a new message
      lastReceivedTick =  newTick;
      userCommand = newUserCommand;
      lastUserCommand = newUserCommand;
      savedTrimCommands = trimCommands;
      updatesSinceLastTick = 0;
      savedEnableTracking = enableTracking;
   else
       updatesSinceLastTick = updatesSinceLastTick + 1;
   end
else
    updatesSinceLastTick = updatesSinceLastTick + 1;
end

%% If the connection to the drone is lost
if updatesSinceLastTick > maxUpdateDelay
    lastUserCommand = Drone_StateModeType(7);
    userCommand = Drone_StateModeType(7);
    
    %% blink led orange
    if ledCounter < 400
        ledCounter = ledCounter + 1;
    else
        ledCounter = 0;
    end
    if ledCounter < 200
        ledColor = 3;
    else 
        ledColor = 0;
    end
end

== matlab function Drone_Flight_Model_StandAlone_KF_Steady/Safety, Drift, interfacing, pre-flight calibarion/Optical Flow/Optical Flow/Template Matching/Hold X Frame/MATLAB Function ==
  data: currentFrame input uint8; referenceFrame output; heldFrame input uint8; flow input
function referenceFrame  = holdFrame(currentFrame,heldFrame,flow)

%% This MATLAB function block holds the T frame untill movement is detected
% If the T frame were updated every step, slow movements would not be
% registered. By holding the frame movement can be measured over multiple
% frames.

if (flow ==0)
    referenceFrame = heldFrame;
else
    referenceFrame = currentFrame;
end

== matlab function Drone_Flight_Model_StandAlone_KF_Steady/Safety, Drift, interfacing, pre-flight calibarion/Optical Flow/Optical Flow/Drone State Correction ==
  data: droneX input; droneY input; droneZ input; trueX output; roll input; pitch input; trueY output; trueZ output
function [trueX, trueY, trueZ]  = inducedDroneStates(droneX, droneY, droneZ, roll, pitch)


pitchR = [cosd(pitch), 0,      -sind(pitch);
            0,         1,       0;
         sind(pitch), 0,       cosd(pitch)];
rollR = [1,     0,              0;
         0,     cosd(roll),     sind(roll);
         0,     -sind(roll),     cosd(roll)];

trueXYZ = pitchR * rollR * [droneX;droneY;droneZ];
trueX = trueXYZ(1);
trueY = trueXYZ(2);
trueZ = trueXYZ(3);

== matlab function Drone_Flight_Model_StandAlone_KF_Steady/Safety, Drift, interfacing, pre-flight calibarion/Zdot transform/Rotation matrix/Rotm in euler ==
  data: alpha input size=3,1; Rbv output size=3,3
function Rbv = fcn(alpha)
Rbv = [1,0,0;0,cos(alpha(1)),sin(alpha(1));0,-sin(alpha(1)),cos(alpha(1))]*...
      [cos(alpha(2)),0,-sin(alpha(2));0,1,0;sin(alpha(2)),0,cos(alpha(2))]*...
      [cos(alpha(3)),sin(alpha(3)),0;-sin(alpha(3)),cos(alpha(3)),0;0,0,1];

== matlab function Drone_Flight_Model_StandAlone_KF_Steady/Take-Off, Landing, Safety, Motor drivers/AR Drone Motors/MotorMixing/Newton To PWM ==
  data: thrustIn input; PWM output; dronePowerScaling parameter
function PWM = newtonToPWM(thrustIn, dronePowerScaling)

%% Base parameters for PWM to Thrust quadratic fit a*x^2 + b*x + c
% Apply drone power scaling to match the base fit between different drones
a = 0.0001116 * dronePowerScaling;
b = 0.005502 * dronePowerScaling;
c = 0.1036 * dronePowerScaling;

%% Compute desired PWM by inverting the quadratic relationship
d = b * b - 4 * a * (c - thrustIn);
PWM = 0 * thrustIn;
% Ensure no imaginary numbers are computed and PWM doesnt become negative
if d > 0 
    candidatePWM = (-b + sqrt(d))/(2 * a);
    if candidatePWM > 0        
        PWM = candidatePWM;
    end
end

== matlab function Drone_Flight_Model_StandAlone_KF_Steady/Safety, Drift, interfacing, pre-flight calibarion/Drone TO PC UDP IO/Gather Data and transfer rates/Prolong flag failure ==
  data: flags input; prolongedFlags output
function prolongedFlags = prolong(flags)

persistent checksumCounter;
persistent resetCounter;
if (isempty(checksumCounter) || isempty(resetCounter))
    resetCounter = 0;
    checksumCounter = 0;
end

holdLength = 400; % ticks

%% prolong if checksum == 0 or resetflag  == 1
prolongedFlags = flags;
% checksum
if flags(1) == 0 || checksumCounter > 0
    prolongedFlags(1) = 0;
    if checksumCounter == 0
        checksumCounter = holdLength
    else
        checksumCounter = checksumCounter - 1;
    end
end

% reset
if flags(2) == 1 || resetCounter > 0
    prolongedFlags(2) = 1;
    if resetCounter == 0
        resetCounter = holdLength
    else
        resetCounter = resetCounter - 1;
    end
end

== matlab function Drone_Flight_Model_StandAlone_KF_Steady/Sensors, Calibration, Raw state computation/RemovePeaks ==
  data: rawHeight input; filteredHeight output; peakThreshold parameter; peakHeightCounterThreshold parameter
function filteredHeight = removePeaks(rawHeight, peakThreshold, peakHeightCounterThreshold)

persistent validHeight
if isempty(validHeight)
    validHeight = rawHeight;
end
persistent peakHeightCounter
if isempty(peakHeightCounter)
    peakHeightCounter = 0;
end

% If the new rawheight does not differ too much it a correct measurement
if abs(rawHeight - validHeight) < peakThreshold
    validHeight = rawHeight;
    peakHeightCounter = 0;
else
    % if the new rawheight does differ a lot but keeps being different for
    % a long time, update the validheight anyway
    peakHeightCounter = peakHeightCounter + 1;
    if (peakHeightCounter > peakHeightCounterThreshold)
        validHeight = rawHeight;
        peakHeightCounter = 0;
    end
end

filteredHeight = validHeight;

== matlab function Drone_Flight_Model_StandAlone_KF_Steady/Sensors, Calibration, Raw state computation/IMU Data Acquisition, Validation, Calibration and Initialization/Measurement Verification and Calibration/Measurement calibration correction/MATLAB Function ==
  data: Ultrasound_Measure input; processed_Ultrasound output
function processed_Ultrasound = removePeak(Ultrasound_Measure)
%#codegen

peakThreshold = 2^15;

persistent validMeasurement
if isempty(validMeasurement)
    validMeasurement = 880;
end

% If the data is a seperator peak
if Ultrasound_Measure >= peakThreshold
    Ultrasound_Measure = Ultrasound_Measure - peakThreshold;
end
% If the data is greater than 880 (minimum usefull lookup table
% breakpoint)
if Ultrasound_Measure > 880
    validMeasurement = Ultrasound_Measure;
end

processed_Ultrasound = validMeasurement;

== matlab function Drone_Flight_Model_StandAlone_KF_Steady/Safety, Drift, interfacing, pre-flight calibarion/Reference State/MATLAB Function ==
  data: x output; defaultHeight input; y output; remoteControl input; trimCommands input; z output; roll output; pitch output; yaw output; drone_StateModeType input
function [x,y,z,roll,pitch,yaw] = processInput(defaultHeight, remoteControl, trimCommands, drone_StateModeType)

persistent dZ;
if isempty(dZ)
    dZ = 0;
end
persistent dY;
if isempty(dY)
    dY = 0;
end
persistent dX;
if isempty(dX)
    dX = 0;
end
persistent dYaw;
if isempty(dYaw)
    dYaw = 0;
end

xRate = 0.5;
yRate = 0.5;
zRate = 0.5;

yawRate = 0.25;

pitch = trimCommands(1);
roll = trimCommands(2);


switch remoteControl
    case 1
        dZ = dZ + zRate;
    case 2
        dZ = dZ - zRate;
    case 3
        dY = dY + yRate;
    case 4
        dY = dY - yRate;
    case 5
        dX = dX + xRate;
    case 6
        dX = dX - xRate;
    case 7
        dYaw = dYaw + yawRate;
    case 8
        dYaw = dYaw - yawRate;
    otherwise
end

% reset all user values if the drone is in the 'WaitForHost' state
if drone_StateModeType == Drone_StateModeType(1)
    dX = 0;
    dY = 0;
    dZ = 0;
    dYaw = 0;
end

x = dX;
y = dY;
z = defaultHeight + dZ;
yaw = dYaw;

== matlab function Drone_Flight_Model_StandAlone_KF_Steady/Safety, Drift, interfacing, pre-flight calibarion/Optical Flow/Optical Flow/Template Matching/Crop Image1 ==
  data: fullFrame input; croppedFrame output
function croppedFrame = CropImage(fullFrame)

%% Template matching works by pixel shifting a smaller image within the full image
% Exhaustive template matching will compute all possible pixel shifts.
% Because of this the cropAmount influences the computation time
% quadratically. A small crop amount increases the computation speed but
% also limits the maximum detectable pixel shift between frames. 
% Three step template matching also has increasing computational time with
% increasing cropAmount, but much less so than the exhaustive method.
cropAmount = 7;
%% Maximizing camera FPS
% Doubling the camera FPS doubles the computation time but also means you 
% can halve the cropAmount and still detect the same velocity range, which 
% reduces the computational time up to a factor 4.
%% FPS limitations
% Using a very high fps means that slow drone movements will not lead to
% significant enough displacement between images. This means that slow
% drift is not detected. Holding the reference frame untill movement is
% deteced is a way around this.


[row, col] = size(fullFrame);
croppedFrame = fullFrame(1 + cropAmount : row - cropAmount, 1 + cropAmount : col - cropAmount);
% croppedFrame = fullFrame(1 + cropAmount : row - cropAmount, 1 : col);

== matlab function Drone_Flight_Model_StandAlone_KF_Steady/Safety, Drift, interfacing, pre-flight calibarion/Drone TO PC UDP IO/Gather Data and transfer rates/MATLAB Function ==
  data: dataToStore input
function storeDataOnDrone(dataToStore)

% the program uses the base dir as working dir while ftp starts from
% /update

fileName = 'update/logData.csv';

persistent fileID
if isempty(fileID)
    fileID = fopen(fileName,'a');
end

formatSpec = ['%f, %f, %f, %f, %f, %f, %f, %f, %f, %f, %f, %f, %f, %f, %f, %f, %f, %f, %f, %f, %f, %f, %f, %f, %f, %f, %f, %f, %f, %f, %f, %f, %f' char(10)...
    '%f, %f, %f, %f, %f, %f, %f, %f, %f, %f, %f, %f, %f, %f, %f, %f, %f, %f, %f, %f, %f, %f, %f, %f, %f, %f, %f, %f, %f, %f, %f, %f, %f' char(10)];
fprintf(fileID,formatSpec,dataToStore(1),dataToStore(2),dataToStore(3),dataToStore(4),dataToStore(5),dataToStore(6),...
    dataToStore(7),dataToStore(8),dataToStore(9),dataToStore(10),dataToStore(11),dataToStore(12),dataToStore(13),...
    dataToStore(14),dataToStore(15),dataToStore(16),dataToStore(17),dataToStore(18),dataToStore(19),dataToStore(20),...
    dataToStore(21),dataToStore(22),dataToStore(23),dataToStore(24),dataToStore(25),dataToStore(26),dataToStore(27),...
    dataToStore(28),dataToStore(29),dataToStore(30),dataToStore(31),dataToStore(32),dataToStore(33),dataToStore(34),...
    dataToStore(35),dataToStore(36),dataToStore(37),dataToStore(38),dataToStore(39),dataToStore(40),dataToStore(41),...
    dataToStore(42),dataToStore(43),dataToStore(44),dataToStore(45),dataToStore(46),dataToStore(47),dataToStore(48),...
    dataToStore(49),dataToStore(50),dataToStore(51),dataToStore(52),dataToStore(53),dataToStore(54),dataToStore(55),...
    dataToStore(56),dataToStore(57),dataToStore(58),dataToStore(59),dataToStore(60),dataToStore(61),dataToStore(62),...
    dataToStore(63),dataToStore(64),dataToStore(65),dataToStore(66));

% format the output into csv (comma seperated values)
% % % THIS DOES NOT WORK BECAUSE CODE GEN DOESNT SUPPORT ARRAY FORMATSPECS
% % fprintf(fileID,'%f, ',dataToStore(1:end-1));
% % fprintf(fileID,['%f' char(10)],dataToStore(end)); % add a newline character

== matlab function Drone_Flight_Model_StandAlone_KF_Steady/Take-Off, Landing, Safety, Motor drivers/Motor Cutoff//Initialize Controller/MATLAB Function ==
  data: hoverControls input; motorControls output; droneState input
function motorControls = motorControlOutput(hoverControls, droneState)

motorControls = [0; 0; 0; 0];

if (droneState == Drone_StateModeType.Landing_RampDown || ...
        droneState == Drone_StateModeType.Landing_Descent || ...
        droneState == Drone_StateModeType.Drift_Compensated_Flight || ...
        droneState == Drone_StateModeType.Object_Tracking_Flight)
    
   motorControls = hoverControls;
end
